simulink model "MPC_RL_H2DF"  (R2023a)
settings: Solver=FixedStepAuto  StartTime=0.0  StopTime=inf  FixedStep=Ts  RelTol=1e-3
model workspace (MAT data in the model file):
  enable_IMEP_noise = 100
  enable_IMEP_offset = 1
values from neighbouring files (symbols this model uses):
  C2C_NMPC = init_C2C_NMPC_H2DF(C2C_NMPC.expdata)    [init_H2DFRL_GRU.m]
  LowerLimit = ([0.17e-3;350;-5;1e-3] - C2C_NMPC.Normalization.controls.mean)./(C2C_NMPC.Normalization.controls.std)    [init_H2DFRL_GRU.m]
  Ts = 0.08    [init_H2DFRL_GRU.m]
  UpperLimit = ([0.5e-3;900;2;5.5e-3] - C2C_NMPC.Normalization.controls.mean)./(C2C_NMPC.Normalization.controls.std)    [init_H2DFRL_GRU.m]
undefined symbols (not defined in the file or in its folder): CA50_offset, DiscIntNeverNeededParam, enable_CA50_noise, enable_CA50_offset, IMEP_offset
libraries: simulink x15, matrix_library x6, dspsigattribs x2, slctrlblks x2, statsLibrary x1, rllib x1
(part 3 of 4)

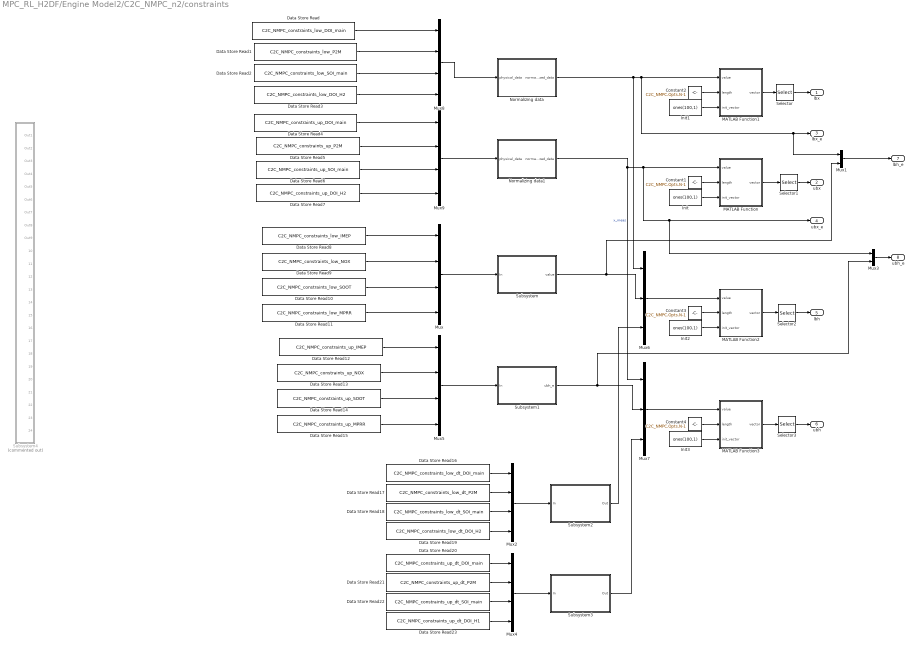
== system MPC_RL_H2DF/Engine Model2/C2C_NMPC_n2/constraints ==
  Constant{1..4} (4 alike) : Constant  Value=C2C_NMPC.Opts.N-1
  Data Store Read : DataStoreRead  DataStoreName=C2C_NMPC_constraints_low_DOI_main  IndexOptions=Index vector (dialog)  Indices=1  OutputSizes=1
  Data Store Read1 : DataStoreRead  DataStoreName=C2C_NMPC_constraints_low_P2M  IndexOptions=Index vector (dialog)  Indices=1  OutputSizes=1
  Data Store Read10 : DataStoreRead  DataStoreName=C2C_NMPC_constraints_low_SOOT  IndexOptions=Index vector (dialog)  Indices=1  OutputSizes=1
  Data Store Read11 : DataStoreRead  DataStoreName=C2C_NMPC_constraints_low_MPRR  IndexOptions=Index vector (dialog)  Indices=1  OutputSizes=1
  Data Store Read12 : DataStoreRead  DataStoreName=C2C_NMPC_constraints_up_IMEP  IndexOptions=Index vector (dialog)  Indices=1  OutputSizes=1
  Data Store Read13 : DataStoreRead  DataStoreName=C2C_NMPC_constraints_up_NOX  IndexOptions=Index vector (dialog)  Indices=1  OutputSizes=1
  Data Store Read14 : DataStoreRead  DataStoreName=C2C_NMPC_constraints_up_SOOT  IndexOptions=Index vector (dialog)  Indices=1  OutputSizes=1
  Data Store Read15 : DataStoreRead  DataStoreName=C2C_NMPC_constraints_up_MPRR  IndexOptions=Index vector (dialog)  Indices=1  OutputSizes=1
  Data Store Read16 : DataStoreRead  DataStoreName=C2C_NMPC_constraints_low_dt_DOI_main  IndexOptions=Index vector (dialog)  Indices=1  OutputSizes=1
  Data Store Read17 : DataStoreRead  DataStoreName=C2C_NMPC_constraints_low_dt_P2M  IndexOptions=Index vector (dialog)  Indices=1  OutputSizes=1
  Data Store Read18 : DataStoreRead  DataStoreName=C2C_NMPC_constraints_low_dt_SOI_main  IndexOptions=Index vector (dialog)  Indices=1  OutputSizes=1
  Data Store Read19 : DataStoreRead  DataStoreName=C2C_NMPC_constraints_low_dt_DOI_H2  IndexOptions=Index vector (dialog)  Indices=1  OutputSizes=1
  Data Store Read2 : DataStoreRead  DataStoreName=C2C_NMPC_constraints_low_SOI_main  IndexOptions=Index vector (dialog)  Indices=1  OutputSizes=1
  Data Store Read20 : DataStoreRead  DataStoreName=C2C_NMPC_constraints_up_dt_DOI_main  IndexOptions=Index vector (dialog)  Indices=1  OutputSizes=1
  Data Store Read21 : DataStoreRead  DataStoreName=C2C_NMPC_constraints_up_dt_P2M  IndexOptions=Index vector (dialog)  Indices=1  OutputSizes=1
  Data Store Read22 : DataStoreRead  DataStoreName=C2C_NMPC_constraints_up_dt_SOI_main  IndexOptions=Index vector (dialog)  Indices=1  OutputSizes=1
  Data Store Read23 : DataStoreRead  DataStoreName=C2C_NMPC_constraints_up_dt_DOI_H1  IndexOptions=Index vector (dialog)  Indices=1  OutputSizes=1
  Data Store Read3 : DataStoreRead  DataStoreName=C2C_NMPC_constraints_low_DOI_H2  IndexOptions=Index vector (dialog)  Indices=1  OutputSizes=1
  Data Store Read4 : DataStoreRead  DataStoreName=C2C_NMPC_constraints_up_DOI_main  IndexOptions=Index vector (dialog)  Indices=1  OutputSizes=1
  Data Store Read5 : DataStoreRead  DataStoreName=C2C_NMPC_constraints_up_P2M  IndexOptions=Index vector (dialog)  Indices=1  OutputSizes=1
  Data Store Read6 : DataStoreRead  DataStoreName=C2C_NMPC_constraints_up_SOI_main  IndexOptions=Index vector (dialog)  Indices=1  OutputSizes=1
  Data Store Read7 : DataStoreRead  DataStoreName=C2C_NMPC_constraints_up_DOI_H2  IndexOptions=Index vector (dialog)  Indices=1  OutputSizes=1
  Data Store Read8 : DataStoreRead  DataStoreName=C2C_NMPC_constraints_low_IMEP  IndexOptions=Index vector (dialog)  Indices=1  OutputSizes=1
  Data Store Read9 : DataStoreRead  DataStoreName=C2C_NMPC_constraints_low_NOX  IndexOptions=Index vector (dialog)  Indices=1  OutputSizes=1
  Init{,1..3} (4 alike) : Constant  Value=ones(100,1)
  MATLAB Function : MATLAB Function  TreatAsAtomicUnit=on
  MATLAB Function1 : MATLAB Function  TreatAsAtomicUnit=on
  MATLAB Function2 : MATLAB Function  TreatAsAtomicUnit=on
  MATLAB Function3 : MATLAB Function  TreatAsAtomicUnit=on
  Mux{,2,4..5,8..9} (6 alike) : Mux
  Mux1 : Mux  Inputs=2
  Mux3 : Mux  Inputs=2
  Mux6 : Mux  Inputs=3
  Mux7 : Mux  Inputs=3
  Normalizing data : Subsystem
  Normalizing data1 : Subsystem
  Selector : Selector  IndexOptions=Index vector (dialog)  Indices=1:((C2C_NMPC.Opts.N-1)*C2C_NMPC.Dims.n_controls)  OutputSizes=1
  Selector1 : Selector  IndexOptions=Index vector (dialog)  Indices=1:((C2C_NMPC.Opts.N-1)*C2C_NMPC.Dims.n_controls)  OutputSizes=1
  Selector2 : Selector  IndexOptions=Index vector (dialog)  Indices=1:((C2C_NMPC.Opts.N)*(C2C_NMPC.Dims.n_outputs + C2C_NMPC.Dims.n_controls +C2C_NMPC.Dims.n_controls))  OutputSizes=1
  Selector3 : Selector  IndexOptions=Index vector (dialog)  Indices=1:((C2C_NMPC.Opts.N)*(C2C_NMPC.Dims.n_outputs + C2C_NMPC.Dims.n_controls +C2C_NMPC.Dims.n_controls))  OutputSizes=1
  Subsystem : Subsystem
  Subsystem1 : Subsystem
  Subsystem2 : Subsystem
  Subsystem3 : Subsystem
  Subsystem4 : Subsystem  Commented=on
  lbx : Outport
  ubx : Outport  Port=2
  lbx_e : Outport  Port=3
  ubx_e : Outport  Port=4
  lbh : Outport  Port=5
  ubh : Outport  Port=6
  lbh_e : Outport  Port=7
  ubh_e : Outport  Port=8
  wires:
  Mux/1 -> Subsystem/1(In)
  Mux5/1 -> Subsystem1/1(In)
  Mux2/1 -> Subsystem2/1(In)
  Mux4/1 -> Subsystem3/1(In)
  Init/1 -> MATLAB Function/3(init_vector)
  Constant1/1 -> MATLAB Function/2(length)
  MATLAB Function/1(vector) -> Selector1/1
  MATLAB Function1/1(vector) -> Selector/1
  Constant2/1 -> MATLAB Function1/2(length)
  Init1/1 -> MATLAB Function1/3(init_vector)
  MATLAB Function2/1(vector) -> Selector2/1
  Constant3/1 -> MATLAB Function2/2(length)
  Init2/1 -> MATLAB Function2/3(init_vector)
  Subsystem3/1(Out) -> Mux7/3
  Mux6/1 -> MATLAB Function2/1(value)
  Normalizing data/1(normalized_data) -> Mux6/1, Mux1/1, lbx_e/1, MATLAB Function1/1(value)
  Subsystem/1(value) -> Mux1/2, Mux6/2
  Subsystem2/1(Out) -> Mux6/3
  MATLAB Function3/1(vector) -> Selector3/1
  Mux7/1 -> MATLAB Function3/1(value)
  Init3/1 -> MATLAB Function3/3(init_vector)
  Constant4/1 -> MATLAB Function3/2(length)
  Data Store Read3/1 -> Mux8/4
  Data Store Read2/1 -> Mux8/3
  Data Store Read1/1 -> Mux8/2
  Data Store Read/1 -> Mux8/1
  Mux8/1 -> Normalizing data/1(physical_data)
  Selector/1 -> lbx/1
  Data Store Read6/1 -> Mux9/3
  Data Store Read5/1 -> Mux9/2
  Data Store Read4/1 -> Mux9/1
  Mux9/1 -> Normalizing data1/1(physical_data)
  Normalizing data1/1(normalized_data) -> Mux7/1, Mux3/1, ubx_e/1, MATLAB Function/1(value)  "x_meas"
  Data Store Read7/1 -> Mux9/4
  Selector1/1 -> ubx/1
  Selector2/1 -> lbh/1
  Selector3/1 -> ubh/1
  Mux1/1 -> lbh_e/1
  Subsystem1/1(ubh_e) -> Mux3/2, Mux7/2
  Mux3/1 -> ubh_e/1
  Data Store Read8/1 -> Mux/1
  Data Store Read9/1 -> Mux/2
  Data Store Read10/1 -> Mux/3
  Data Store Read11/1 -> Mux/4
  Data Store Read12/1 -> Mux5/1
  Data Store Read13/1 -> Mux5/2
  Data Store Read14/1 -> Mux5/3
  Data Store Read15/1 -> Mux5/4
  Data Store Read16/1 -> Mux2/1
  Data Store Read17/1 -> Mux2/2
  Data Store Read18/1 -> Mux2/3
  Data Store Read19/1 -> Mux2/4
  Data Store Read20/1 -> Mux4/1
  Data Store Read21/1 -> Mux4/2
  Data Store Read22/1 -> Mux4/3
  Data Store Read23/1 -> Mux4/4

== system MPC_RL_H2DF/Engine Model2/C2C_NMPC_n2/cost_function_weights ==
  Create Diagonal Matrix : matrix_library/Create Diagonal Matrix
  Create Diagonal Matrix1 : matrix_library/Create Diagonal Matrix
  Create Diagonal Matrix2 : matrix_library/Create Diagonal Matrix
  Data Store Read : DataStoreRead  DataStoreName=C2C_NMPC_IMEP_Weight  IndexOptions=Index vector (dialog)  Indices=1  OutputSizes=1
  Data Store Read1 : DataStoreRead  DataStoreName=C2C_NMPC_NOX_Weight  IndexOptions=Index vector (dialog)  Indices=1  OutputSizes=1
  Data Store Read10 : DataStoreRead  DataStoreName=C2C_NMPC_Delta_SOI_Main_Weight  IndexOptions=Index vector (dialog)  Indices=1  OutputSizes=1
  Data Store Read11 : DataStoreRead  DataStoreName=C2C_NMPC_Delta_DOI_H2_Weight  IndexOptions=Index vector (dialog)  Indices=1  OutputSizes=1
  Data Store Read12 : DataStoreRead  DataStoreName=C2C_NMPC_alpha  IndexOptions=Index vector (dialog)  Indices=1  OutputSizes=1
  Data Store Read13 : DataStoreRead  DataStoreName=C2C_NMPC_beta  IndexOptions=Index vector (dialog)  Indices=1  OutputSizes=1
  Data Store Read14 : DataStoreRead  DataStoreName=C2C_NMPC_gamma  IndexOptions=Index vector (dialog)  Indices=1  OutputSizes=1
  Data Store Read2 : DataStoreRead  DataStoreName=C2C_NMPC_SOOT_Weight  IndexOptions=Index vector (dialog)  Indices=1  OutputSizes=1
  Data Store Read3 : DataStoreRead  DataStoreName=C2C_NMPC_MPRR_Weight  IndexOptions=Index vector (dialog)  Indices=1  OutputSizes=1
  Data Store Read4 : DataStoreRead  DataStoreName=C2C_NMPC_DOI_Main_Weight  IndexOptions=Index vector (dialog)  Indices=1  OutputSizes=1
  Data Store Read5 : DataStoreRead  DataStoreName=C2C_NMPC_P2M_Weight  IndexOptions=Index vector (dialog)  Indices=1  OutputSizes=1
  Data Store Read6 : DataStoreRead  DataStoreName=C2C_NMPC_SOI_Main_Weight  IndexOptions=Index vector (dialog)  Indices=1  OutputSizes=1
  Data Store Read7 : DataStoreRead  DataStoreName=C2C_NMPC_DOI_H2_Weight  IndexOptions=Index vector (dialog)  Indices=1  OutputSizes=1
  Data Store Read8 : DataStoreRead  DataStoreName=C2C_NMPC_Delta_DOI_Main_Weight  IndexOptions=Index vector (dialog)  Indices=1  OutputSizes=1
  Data Store Read9 : DataStoreRead  DataStoreName=C2C_NMPC_Delta_P2M_Weight  IndexOptions=Index vector (dialog)  Indices=1  OutputSizes=1
  Mux : Mux
  Mux2 : Mux
  Mux3 : Mux
  Normalize 0 to 1 : Subsystem
  Product : Product
  Product1 : Product
  Product2 : Product
  alpha : Gain  Commented=on
  beta : Gain  Commented=on  Gain=0.001
  blkdiag Function : MATLAB Function  TreatAsAtomicUnit=on
  blkdiag Function1 : MATLAB Function  TreatAsAtomicUnit=on
  gamma1 : Gain  Commented=on  Gain=2
  cost_W : Outport
  cost_W_e : Outport  Port=2
  wires:
  blkdiag Function/1(y) -> cost_W/1
  Create Diagonal Matrix2/1 -> blkdiag Function/3(u3)
  Product2/1 -> Create Diagonal Matrix2/1
  Create Diagonal Matrix1/1 -> blkdiag Function1/2(u2), blkdiag Function/2(u2)
  Data Store Read7/1 -> Mux3/4
  Data Store Read4/1 -> Mux3/1
  Data Store Read6/1 -> Mux3/3
  Data Store Read5/1 -> Mux3/2
  Mux3/1 -> Product1/1
  Product1/1 -> Create Diagonal Matrix/1
  Product/1 -> Create Diagonal Matrix1/1
  Mux/1 -> Product/1
  Data Store Read1/1 -> Mux/2
  Data Store Read/1 -> Mux/1
  Data Store Read3/1 -> Mux/4
  Data Store Read2/1 -> Mux/3
  Create Diagonal Matrix/1 -> blkdiag Function1/1(u1), blkdiag Function/1(u1)
  Data Store Read8/1 -> Mux2/1
  Data Store Read9/1 -> Mux2/2
  Data Store Read10/1 -> Mux2/3
  Data Store Read11/1 -> Mux2/4
  Data Store Read12/1 -> Product/2
  Data Store Read13/1 -> Product1/2
  Data Store Read14/1 -> Product2/2
  Mux2/1 -> Product2/1
  blkdiag Function1/1(y) -> cost_W_e/1

== system MPC_RL_H2DF/Engine Model2/offset_and_noise/CA50_generation ==
  CA50_in : Inport
  Add : Sum
  Add1 : Sum
  Band-Limited White Noise : simulink/Sources/Band-Limited White Noise  Cov=0.01  Ts=1  seed=[23341]
  Constant1 : Constant  Value=CA50_offset
  Constant2 : Constant  Value=0
  Constant3 : Constant  Value=enable_CA50_noise
  Constant4 : Constant  Value=0
  Constant5 : Constant  Value=enable_CA50_offset
  Switch1 : Switch  Criteria=u2 > Threshold  SaturateOnIntegerOverflow=off  InputSameDT=off
  Switch2 : Switch  Criteria=u2 > Threshold  SaturateOnIntegerOverflow=off  InputSameDT=off
  denormalizing_CA50 : Subsystem
  normalizing_CA50 : Subsystem
  CA50_out : Outport
  wires:
  Add/1 -> Add1/2
  Switch1/1 -> Add1/1
  Constant4/1 -> Switch1/3
  Constant3/1 -> Switch1/2
  Band-Limited White Noise/1 -> Switch1/1
  CA50_in/1 -> denormalizing_CA50/1(CA50_in)
  denormalizing_CA50/1(CA50) -> Add/2
  Switch2/1 -> Add/1
  Constant1/1 -> Switch2/1
  Constant5/1 -> Switch2/2
  Constant2/1 -> Switch2/3
  normalizing_CA50/1(CA50_out) -> CA50_out/1
  Add1/1 -> normalizing_CA50/1(CA50)

== system MPC_RL_H2DF/Engine Model2/offset_and_noise/IMEP_generation ==
  IMEP_in : Inport
  Add : Sum
  Add1 : Sum
  Band-Limited White Noise : simulink/Sources/Band-Limited White Noise  Cov=0.01  Ts=1  seed=[23341]
  Constant1 : Constant  Value=IMEP_offset
  Constant2 : Constant  Value=0
  Constant3 : Constant  Value=enable_IMEP_noise
  Constant4 : Constant  Value=0
  Constant5 : Constant  Value=enable_IMEP_offset
  Switch1 : Switch  Criteria=u2 > Threshold  SaturateOnIntegerOverflow=off  InputSameDT=off
  Switch2 : Switch  Criteria=u2 > Threshold  SaturateOnIntegerOverflow=off  InputSameDT=off
  denormalizing_IMEP : Subsystem
  normalizing_IMEP : Subsystem
  IMEP_out : Outport
  wires:
  Add/1 -> Add1/2
  Switch1/1 -> Add1/1
  Constant4/1 -> Switch1/3
  Constant3/1 -> Switch1/2
  Band-Limited White Noise/1 -> Switch1/1
  IMEP_in/1 -> denormalizing_IMEP/1(IMEP_in)
  denormalizing_IMEP/1(IMEP) -> Add/2
  Switch2/1 -> Add/1
  Constant1/1 -> Switch2/1
  Constant5/1 -> Switch2/2
  Constant2/1 -> Switch2/3
  normalizing_IMEP/1(IMEP_out) -> IMEP_out/1
  Add1/1 -> normalizing_IMEP/1(IMEP)

== system MPC_RL_H2DF/Engine Model2/offset_and_noise1/IMEP_generation ==
  IMEP_in : Inport
  Add : Sum
  Add1 : Sum
  Add2 : Sum  Inputs=+-
  Band-Limited White Noise : simulink/Sources/Band-Limited White Noise  Cov=0.1  Ts=Ts  seed=[23341]
  Constant1 : Constant  Commented=on  Value=IMEP_offset
  Constant2 : Constant  Value=0
  Constant3 : Constant  Value=enable_IMEP_noise
  Constant4 : Constant  Value=0
  Constant5 : Constant  Value=enable_IMEP_offset
  Constant6 : Constant  Value=0
  Display : Display
  Gain : Gain  Gain=10000
  Scope : Scope  NumInputPorts=2
  Scope1 : Scope
  Switch1 : Switch  Criteria=u2 > Threshold  SaturateOnIntegerOverflow=off  InputSameDT=off
  Switch2 : Switch  Criteria=u2 > Threshold  SaturateOnIntegerOverflow=off  InputSameDT=off
  denormalizing_IMEP : Subsystem
  normalizing_IMEP : Subsystem
  IMEP_out : Outport
  wires:
  Add/1 -> Add1/2
  Switch1/1 -> Display/1, Add1/1
  Constant4/1 -> Switch1/3
  Constant3/1 -> Switch1/2
  Band-Limited White Noise/1 -> Gain/1
  denormalizing_IMEP/1(IMEP) -> Add/2
  Switch2/1 -> Add/1
  Constant5/1 -> Switch2/2
  Constant2/1 -> Switch2/3
  normalizing_IMEP/1(IMEP_out) -> IMEP_out/1
  Add1/1 -> Add2/1, Scope/2, normalizing_IMEP/1(IMEP)
  Constant6/1 -> Switch2/1
  Gain/1 -> Switch1/1
  IMEP_in/1 -> Scope/1, Add2/2, denormalizing_IMEP/1(IMEP_in)
  Add2/1 -> Scope1/1

== system MPC_RL_H2DF/Engine Model2/offset_and_noise2/IMEP_generation ==
  IMEP_in : Inport
  Add : Sum
  Add1 : Sum
  Add2 : Sum  Inputs=+-
  Band-Limited White Noise : simulink/Sources/Band-Limited White Noise  Cov=0.1  Ts=Ts  seed=[23341]
  Constant1 : Constant  Commented=on  Value=IMEP_offset
  Constant2 : Constant  Value=0
  Constant3 : Constant  Value=enable_IMEP_noise
  Constant4 : Constant  Value=0
  Constant5 : Constant  Value=enable_IMEP_offset
  Constant6 : Constant  Value=0
  Display : Display
  Gain : Gain  Gain=10000
  Scope : Scope  NumInputPorts=2
  Scope1 : Scope
  Switch1 : Switch  Criteria=u2 > Threshold  SaturateOnIntegerOverflow=off  InputSameDT=off
  Switch2 : Switch  Criteria=u2 > Threshold  SaturateOnIntegerOverflow=off  InputSameDT=off
  denormalizing_IMEP : Subsystem
  normalizing_IMEP : Subsystem
  IMEP_out : Outport
  wires:
  Add/1 -> Add1/2
  Switch1/1 -> Display/1, Add1/1
  Constant4/1 -> Switch1/3
  Constant3/1 -> Switch1/2
  Band-Limited White Noise/1 -> Gain/1
  denormalizing_IMEP/1(IMEP) -> Add/2
  Switch2/1 -> Add/1
  Constant5/1 -> Switch2/2
  Constant2/1 -> Switch2/3
  normalizing_IMEP/1(IMEP_out) -> IMEP_out/1
  Add1/1 -> Add2/1, Scope/2, normalizing_IMEP/1(IMEP)
  Constant6/1 -> Switch2/1
  Gain/1 -> Switch1/1
  IMEP_in/1 -> Scope/1, Add2/2, denormalizing_IMEP/1(IMEP_in)
  Add2/1 -> Scope1/1

== system MPC_RL_H2DF/Engine Model2/offset_and_noise3/IMEP_generation ==
  IMEP_in : Inport
  Add : Sum
  Add1 : Sum
  Add2 : Sum  Inputs=+-
  Band-Limited White Noise : simulink/Sources/Band-Limited White Noise  Cov=0.1  Ts=Ts  seed=[23341]
  Constant1 : Constant  Commented=on  Value=IMEP_offset
  Constant2 : Constant  Value=0
  Constant3 : Constant  Value=enable_IMEP_noise
  Constant4 : Constant  Value=0
  Constant5 : Constant  Value=enable_IMEP_offset
  Constant6 : Constant  Value=0
  Display : Display
  Gain : Gain  Gain=10000
  Scope : Scope  NumInputPorts=2
  Scope1 : Scope
  Switch1 : Switch  Criteria=u2 > Threshold  SaturateOnIntegerOverflow=off  InputSameDT=off
  Switch2 : Switch  Criteria=u2 > Threshold  SaturateOnIntegerOverflow=off  InputSameDT=off
  denormalizing_IMEP : Subsystem
  normalizing_IMEP : Subsystem
  IMEP_out : Outport
  wires:
  Add/1 -> Add1/2
  Switch1/1 -> Display/1, Add1/1
  Constant4/1 -> Switch1/3
  Constant3/1 -> Switch1/2
  Band-Limited White Noise/1 -> Gain/1
  denormalizing_IMEP/1(IMEP) -> Add/2
  Switch2/1 -> Add/1
  Constant5/1 -> Switch2/2
  Constant2/1 -> Switch2/3
  normalizing_IMEP/1(IMEP_out) -> IMEP_out/1
  Add1/1 -> Add2/1, Scope/2, normalizing_IMEP/1(IMEP)
  Constant6/1 -> Switch2/1
  Gain/1 -> Switch1/1
  IMEP_in/1 -> Scope/1, Add2/2, denormalizing_IMEP/1(IMEP_in)
  Add2/1 -> Scope1/1

== system MPC_RL_H2DF/Engine Model2/reference1/Subsystem4 ==
  C2C_NMPC_constraints_low_dt_DOI_H1 : Constant  Value=-1e6
  C2C_NMPC_constraints_low_dt_DOI_main1 : Constant  Value=-1e6
  C2C_NMPC_constraints_low_dt_P2M1 : Constant  Value=-1e6
  C2C_NMPC_constraints_low_dt_SOI_main1 : Constant  Value=-1e6
  C2C_NMPC_constraints_up_dt_DOI_H2 : Constant  Value=1e6
  C2C_NMPC_constraints_up_dt_DOI_main1 : Constant  Value=1e6
  C2C_NMPC_constraints_up_dt_P2M1 : Constant  Value=1e6
  C2C_NMPC_constraints_up_dt_SOI_main1 : Constant  Value=1e6
  Data Store Write16 : DataStoreWrite  DataStoreName=C2C_NMPC_constraints_low_dt_DOI_main  IndexOptions=Index vector (dialog)  Indices=1  OutputSizes=1
  Data Store Write17 : DataStoreWrite  DataStoreName=C2C_NMPC_constraints_low_dt_P2M  IndexOptions=Index vector (dialog)  Indices=1  OutputSizes=1
  Data Store Write18 : DataStoreWrite  DataStoreName=C2C_NMPC_constraints_low_dt_SOI_main  IndexOptions=Index vector (dialog)  Indices=1  OutputSizes=1
  Data Store Write19 : DataStoreWrite  DataStoreName=C2C_NMPC_constraints_low_dt_DOI_H2  IndexOptions=Index vector (dialog)  Indices=1  OutputSizes=1
  Data Store Write20 : DataStoreWrite  DataStoreName=C2C_NMPC_constraints_up_dt_DOI_main  IndexOptions=Index vector (dialog)  Indices=1  OutputSizes=1
  Data Store Write21 : DataStoreWrite  DataStoreName=C2C_NMPC_constraints_up_dt_P2M  IndexOptions=Index vector (dialog)  Indices=1  OutputSizes=1
  Data Store Write22 : DataStoreWrite  DataStoreName=C2C_NMPC_constraints_up_dt_SOI_main  IndexOptions=Index vector (dialog)  Indices=1  OutputSizes=1
  Data Store Write23 : DataStoreWrite  DataStoreName=C2C_NMPC_constraints_up_dt_DOI_H1  IndexOptions=Index vector (dialog)  Indices=1  OutputSizes=1
  wires:
  C2C_NMPC_constraints_up_dt_P2M1/1 -> Data Store Write21/1
  C2C_NMPC_constraints_low_dt_SOI_main1/1 -> Data Store Write18/1
  C2C_NMPC_constraints_up_dt_DOI_main1/1 -> Data Store Write20/1
  C2C_NMPC_constraints_low_dt_P2M1/1 -> Data Store Write17/1
  C2C_NMPC_constraints_up_dt_SOI_main1/1 -> Data Store Write22/1
  C2C_NMPC_constraints_low_dt_DOI_main1/1 -> Data Store Write16/1
  C2C_NMPC_constraints_low_dt_DOI_H1/1 -> Data Store Write19/1
  C2C_NMPC_constraints_up_dt_DOI_H2/1 -> Data Store Write23/1

== system MPC_RL_H2DF/Engine Model2/results/denormalizing physical controls and outputs ==
  IMEP_norm : Inport
  NOX_norm : Inport  Port=2
  soot_norm : Inport  Port=3
  MPRR_norm : Inport  Port=4
  DOI_main_norm : Inport  Port=5
  SOI_pre_norm : Inport  Port=6
  SOI_main_norm : Inport  Port=7
  DOI_H2_norm : Inport  Port=8
  Constant : Constant  Value=C2C_NMPC.Normalization.outputs.mean(1)
  Constant1 : Constant  Value=C2C_NMPC.Normalization.controls.mean(4)
  Constant3 : Constant  Value=C2C_NMPC.Normalization.outputs.mean(2)
  Constant4 : Constant  Value=C2C_NMPC.Normalization.outputs.mean(3)
  Constant5 : Constant  Value=C2C_NMPC.Normalization.outputs.mean(4)
  Constant6 : Constant  Value=C2C_NMPC.Normalization.controls.mean(1)
  Constant7 : Constant  Value=C2C_NMPC.Normalization.controls.mean(2)
  Constant8 : Constant  Value=C2C_NMPC.Normalization.controls.mean(3)
  Gain : Gain  Gain=C2C_NMPC.Normalization.outputs.std(1)
  Gain1 : Gain  Gain=C2C_NMPC.Normalization.controls.std(4)
  Gain3 : Gain  Gain=C2C_NMPC.Normalization.outputs.std(2)
  Gain4 : Gain  Gain=C2C_NMPC.Normalization.outputs.std(3)
  Gain5 : Gain  Gain=C2C_NMPC.Normalization.outputs.std(4)
  Gain6 : Gain  Gain=C2C_NMPC.Normalization.controls.std(1)
  Gain7 : Gain  Gain=C2C_NMPC.Normalization.controls.std(2)
  Gain8 : Gain  Gain=C2C_NMPC.Normalization.controls.std(3)
  Sum{1,3..8,10} (8 alike) : Sum  Inputs=|++
  IMEP : Outport
  NOX : Outport  Port=2
  soot : Outport  Port=3
  MPRR : Outport  Port=4
  DOI_main : Outport  Port=5
  SOI_pre : Outport  Port=6
  SOI_main : Outport  Port=7
  DOI_H2 : Outport  Port=8
  wires:
  Gain4/1 -> Sum4/1
  Constant3/1 -> Sum3/2
  Constant4/1 -> Sum4/2
  Gain3/1 -> Sum3/1
  Constant5/1 -> Sum5/2
  Gain5/1 -> Sum5/1
  Constant/1 -> Sum6/2
  Sum3/1 -> NOX/1
  NOX_norm/1 -> Gain3/1
  Sum5/1 -> MPRR/1
  Gain/1 -> Sum6/1
  IMEP_norm/1 -> Gain/1
  Sum6/1 -> IMEP/1
  MPRR_norm/1 -> Gain5/1
  Sum4/1 -> soot/1
  soot_norm/1 -> Gain4/1
  Constant7/1 -> Sum8/2
  Gain8/1 -> Sum10/1
  Constant6/1 -> Sum7/2
  Gain7/1 -> Sum8/1
  Sum10/1 -> SOI_main/1
  DOI_main_norm/1 -> Gain6/1
  Sum7/1 -> DOI_main/1
  Gain6/1 -> Sum7/1
  Sum8/1 -> SOI_pre/1
  Constant8/1 -> Sum10/2
  SOI_main_norm/1 -> Gain8/1
  SOI_pre_norm/1 -> Gain7/1
  DOI_H2_norm/1 -> Gain1/1
  Constant1/1 -> Sum1/2
  Gain1/1 -> Sum1/1
  Sum1/1 -> DOI_H2/1

== system MPC_RL_H2DF/Engine Model2/results/denormalizing reference ==
  IMEP_norm : Inport
  NOX_norm : Inport  Port=2
  soot_norm : Inport  Port=3
  MPRR_norm : Inport  Port=4
  Constant : Constant  Value=C2C_NMPC.Normalization.outputs.mean(1)
  Constant1 : Constant  Value=C2C_NMPC.Normalization.outputs.mean(2)
  Constant2 : Constant  Value=C2C_NMPC.Normalization.outputs.mean(3)
  Constant3 : Constant  Value=C2C_NMPC.Normalization.outputs.mean(4)
  Gain : Gain  Gain=C2C_NMPC.Normalization.outputs.std(1)
  Gain1 : Gain  Gain=C2C_NMPC.Normalization.outputs.std(2)
  Gain2 : Gain  Gain=C2C_NMPC.Normalization.outputs.std(3)
  Gain3 : Gain  Gain=C2C_NMPC.Normalization.outputs.std(4)
  Sum{1..3,5} (4 alike) : Sum  Inputs=|++
  IMEP : Outport
  NOX : Outport  Port=2
  soot : Outport  Port=3
  MPRR : Outport  Port=4
  wires:
  Gain/1 -> Sum5/1
  IMEP_norm/1 -> Gain/1
  Constant/1 -> Sum5/2
  Sum5/1 -> IMEP/1
  Gain1/1 -> Sum1/1
  Constant1/1 -> Sum1/2
  NOX_norm/1 -> Gain1/1
  Sum1/1 -> NOX/1
  Gain2/1 -> Sum2/1
  Constant2/1 -> Sum2/2
  soot_norm/1 -> Gain2/1
  Sum2/1 -> soot/1
  Gain3/1 -> Sum3/1
  Constant3/1 -> Sum3/2
  MPRR_norm/1 -> Gain3/1
  Sum3/1 -> MPRR/1

== system MPC_RL_H2DF/Engine Model2/results1/denormalizing physical controls and outputs ==
  IMEP_norm : Inport
  NOX_norm : Inport  Port=2
  soot_norm : Inport  Port=3
  MPRR_norm : Inport  Port=4
  DOI_main_norm : Inport  Port=5
  SOI_pre_norm : Inport  Port=6
  SOI_main_norm : Inport  Port=7
  DOI_H2_norm : Inport  Port=8
  Constant : Constant  Value=C2C_NMPC.Normalization.outputs.mean(1)
  Constant1 : Constant  Value=C2C_NMPC.Normalization.controls.mean(4)
  Constant3 : Constant  Value=C2C_NMPC.Normalization.outputs.mean(2)
  Constant4 : Constant  Value=C2C_NMPC.Normalization.outputs.mean(3)
  Constant5 : Constant  Value=C2C_NMPC.Normalization.outputs.mean(4)
  Constant6 : Constant  Value=C2C_NMPC.Normalization.controls.mean(1)
  Constant7 : Constant  Value=C2C_NMPC.Normalization.controls.mean(2)
  Constant8 : Constant  Value=C2C_NMPC.Normalization.controls.mean(3)
  Gain : Gain  Gain=C2C_NMPC.Normalization.outputs.std(1)
  Gain1 : Gain  Gain=C2C_NMPC.Normalization.controls.std(4)
  Gain3 : Gain  Gain=C2C_NMPC.Normalization.outputs.std(2)
  Gain4 : Gain  Gain=C2C_NMPC.Normalization.outputs.std(3)
  Gain5 : Gain  Gain=C2C_NMPC.Normalization.outputs.std(4)
  Gain6 : Gain  Gain=C2C_NMPC.Normalization.controls.std(1)
  Gain7 : Gain  Gain=C2C_NMPC.Normalization.controls.std(2)
  Gain8 : Gain  Gain=C2C_NMPC.Normalization.controls.std(3)
  Sum{1,3..8,10} (8 alike) : Sum  Inputs=|++
  IMEP : Outport
  NOX : Outport  Port=2
  soot : Outport  Port=3
  MPRR : Outport  Port=4
  DOI_main : Outport  Port=5
  SOI_pre : Outport  Port=6
  SOI_main : Outport  Port=7
  DOI_H2 : Outport  Port=8
  wires:
  Gain4/1 -> Sum4/1
  Constant3/1 -> Sum3/2
  Constant4/1 -> Sum4/2
  Gain3/1 -> Sum3/1
  Constant5/1 -> Sum5/2
  Gain5/1 -> Sum5/1
  Constant/1 -> Sum6/2
  Sum3/1 -> NOX/1
  NOX_norm/1 -> Gain3/1
  Sum5/1 -> MPRR/1
  Gain/1 -> Sum6/1
  IMEP_norm/1 -> Gain/1
  Sum6/1 -> IMEP/1
  MPRR_norm/1 -> Gain5/1
  Sum4/1 -> soot/1
  soot_norm/1 -> Gain4/1
  Constant7/1 -> Sum8/2
  Gain8/1 -> Sum10/1
  Constant6/1 -> Sum7/2
  Gain7/1 -> Sum8/1
  Sum10/1 -> SOI_main/1
  DOI_main_norm/1 -> Gain6/1
  Sum7/1 -> DOI_main/1
  Gain6/1 -> Sum7/1
  Sum8/1 -> SOI_pre/1
  Constant8/1 -> Sum10/2
  SOI_main_norm/1 -> Gain8/1
  SOI_pre_norm/1 -> Gain7/1
  DOI_H2_norm/1 -> Gain1/1
  Constant1/1 -> Sum1/2
  Gain1/1 -> Sum1/1
  Sum1/1 -> DOI_H2/1

== system MPC_RL_H2DF/Engine Model2/results1/denormalizing reference ==
  IMEP_norm : Inport
  NOX_norm : Inport  Port=2
  soot_norm : Inport  Port=3
  MPRR_norm : Inport  Port=4
  Constant : Constant  Value=C2C_NMPC.Normalization.outputs.mean(1)
  Constant1 : Constant  Value=C2C_NMPC.Normalization.outputs.mean(2)
  Constant2 : Constant  Value=C2C_NMPC.Normalization.outputs.mean(3)
  Constant3 : Constant  Value=C2C_NMPC.Normalization.outputs.mean(4)
  Gain : Gain  Gain=C2C_NMPC.Normalization.outputs.std(1)
  Gain1 : Gain  Gain=C2C_NMPC.Normalization.outputs.std(2)
  Gain2 : Gain  Gain=C2C_NMPC.Normalization.outputs.std(3)
  Gain3 : Gain  Gain=C2C_NMPC.Normalization.outputs.std(4)
  Sum{1..3,5} (4 alike) : Sum  Inputs=|++
  IMEP : Outport
  NOX : Outport  Port=2
  soot : Outport  Port=3
  MPRR : Outport  Port=4
  wires:
  Gain/1 -> Sum5/1
  IMEP_norm/1 -> Gain/1
  Constant/1 -> Sum5/2
  Sum5/1 -> IMEP/1
  Gain1/1 -> Sum1/1
  Constant1/1 -> Sum1/2
  NOX_norm/1 -> Gain1/1
  Sum1/1 -> NOX/1
  Gain2/1 -> Sum2/1
  Constant2/1 -> Sum2/2
  soot_norm/1 -> Gain2/1
  Sum2/1 -> soot/1
  Gain3/1 -> Sum3/1
  Constant3/1 -> Sum3/2
  MPRR_norm/1 -> Gain3/1
  Sum3/1 -> MPRR/1

== system MPC_RL_H2DF/Engine Model2/results2/denormalizing physical controls and outputs ==
  IMEP_norm : Inport
  NOX_norm : Inport  Port=2
  soot_norm : Inport  Port=3
  MPRR_norm : Inport  Port=4
  DOI_main_norm : Inport  Port=5
  SOI_pre_norm : Inport  Port=6
  SOI_main_norm : Inport  Port=7
  DOI_H2_norm : Inport  Port=8
  Constant : Constant  Value=C2C_NMPC.Normalization.outputs.mean(1)
  Constant1 : Constant  Value=C2C_NMPC.Normalization.controls.mean(4)
  Constant3 : Constant  Value=C2C_NMPC.Normalization.outputs.mean(2)
  Constant4 : Constant  Value=C2C_NMPC.Normalization.outputs.mean(3)
  Constant5 : Constant  Value=C2C_NMPC.Normalization.outputs.mean(4)
  Constant6 : Constant  Value=C2C_NMPC.Normalization.controls.mean(1)
  Constant7 : Constant  Value=C2C_NMPC.Normalization.controls.mean(2)
  Constant8 : Constant  Value=C2C_NMPC.Normalization.controls.mean(3)
  Gain : Gain  Gain=C2C_NMPC.Normalization.outputs.std(1)
  Gain1 : Gain  Gain=C2C_NMPC.Normalization.controls.std(4)
  Gain3 : Gain  Gain=C2C_NMPC.Normalization.outputs.std(2)
  Gain4 : Gain  Gain=C2C_NMPC.Normalization.outputs.std(3)
  Gain5 : Gain  Gain=C2C_NMPC.Normalization.outputs.std(4)
  Gain6 : Gain  Gain=C2C_NMPC.Normalization.controls.std(1)
  Gain7 : Gain  Gain=C2C_NMPC.Normalization.controls.std(2)
  Gain8 : Gain  Gain=C2C_NMPC.Normalization.controls.std(3)
  Sum{1,3..8,10} (8 alike) : Sum  Inputs=|++
  IMEP : Outport
  NOX : Outport  Port=2
  soot : Outport  Port=3
  MPRR : Outport  Port=4
  DOI_main : Outport  Port=5
  SOI_pre : Outport  Port=6
  SOI_main : Outport  Port=7
  DOI_H2 : Outport  Port=8
  wires:
  Gain4/1 -> Sum4/1
  Constant3/1 -> Sum3/2
  Constant4/1 -> Sum4/2
  Gain3/1 -> Sum3/1
  Constant5/1 -> Sum5/2
  Gain5/1 -> Sum5/1
  Constant/1 -> Sum6/2
  Sum3/1 -> NOX/1
  NOX_norm/1 -> Gain3/1
  Sum5/1 -> MPRR/1
  Gain/1 -> Sum6/1
  IMEP_norm/1 -> Gain/1
  Sum6/1 -> IMEP/1
  MPRR_norm/1 -> Gain5/1
  Sum4/1 -> soot/1
  soot_norm/1 -> Gain4/1
  Constant7/1 -> Sum8/2
  Gain8/1 -> Sum10/1
  Constant6/1 -> Sum7/2
  Gain7/1 -> Sum8/1
  Sum10/1 -> SOI_main/1
  DOI_main_norm/1 -> Gain6/1
  Sum7/1 -> DOI_main/1
  Gain6/1 -> Sum7/1
  Sum8/1 -> SOI_pre/1
  Constant8/1 -> Sum10/2
  SOI_main_norm/1 -> Gain8/1
  SOI_pre_norm/1 -> Gain7/1
  DOI_H2_norm/1 -> Gain1/1
  Constant1/1 -> Sum1/2
  Gain1/1 -> Sum1/1
  Sum1/1 -> DOI_H2/1

== system MPC_RL_H2DF/Engine Model2/results2/denormalizing reference ==
  IMEP_norm : Inport
  NOX_norm : Inport  Port=2
  soot_norm : Inport  Port=3
  MPRR_norm : Inport  Port=4
  Constant : Constant  Value=C2C_NMPC.Normalization.outputs.mean(1)
  Constant1 : Constant  Value=C2C_NMPC.Normalization.outputs.mean(2)
  Constant2 : Constant  Value=C2C_NMPC.Normalization.outputs.mean(3)
  Constant3 : Constant  Value=C2C_NMPC.Normalization.outputs.mean(4)
  Gain : Gain  Gain=C2C_NMPC.Normalization.outputs.std(1)
  Gain1 : Gain  Gain=C2C_NMPC.Normalization.outputs.std(2)
  Gain2 : Gain  Gain=C2C_NMPC.Normalization.outputs.std(3)
  Gain3 : Gain  Gain=C2C_NMPC.Normalization.outputs.std(4)
  Sum{1..3,5} (4 alike) : Sum  Inputs=|++
  IMEP : Outport
  NOX : Outport  Port=2
  soot : Outport  Port=3
  MPRR : Outport  Port=4
  wires:
  Gain/1 -> Sum5/1
  IMEP_norm/1 -> Gain/1
  Constant/1 -> Sum5/2
  Sum5/1 -> IMEP/1
  Gain1/1 -> Sum1/1
  Constant1/1 -> Sum1/2
  NOX_norm/1 -> Gain1/1
  Sum1/1 -> NOX/1
  Gain2/1 -> Sum2/1
  Constant2/1 -> Sum2/2
  soot_norm/1 -> Gain2/1
  Sum2/1 -> soot/1
  Gain3/1 -> Sum3/1
  Constant3/1 -> Sum3/2
  MPRR_norm/1 -> Gain3/1
  Sum3/1 -> MPRR/1

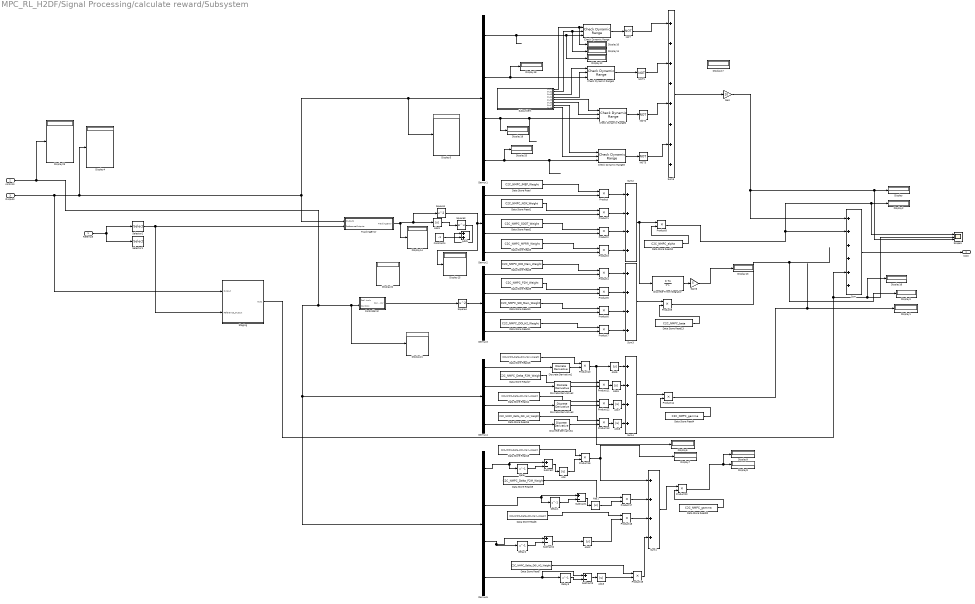
== system MPC_RL_H2DF/Signal Processing/calculate reward/Subsystem ==
  Refernce : Inport
  controls : Inport  Port=2
  Outputs : Inport  Port=3
  Abs{,1..3,5..9} (9 alike) : Abs  SaturateOnIntegerOverflow=off
  Add1 : Sum
  Check Dynamic Range{,1..3} (4 alike) : simulink/Model Verification/Check  Dynamic Range  Description=min < u < max  enabled=off  stopWhenAssertionFail=off  export=on  icon=graphic
  Constant4 : Constant  Value=-1
  ControlError : Subsystem
  Data Store Read : DataStoreRead  DataStoreName=C2C_NMPC_IMEP_Weight  IndexOptions=Index vector (dialog)  Indices=1  OutputSizes=1
  Data Store Read1 : DataStoreRead  DataStoreName=C2C_NMPC_NOX_Weight  IndexOptions=Index vector (dialog)  Indices=1  OutputSizes=1
  Data Store Read10 : DataStoreRead  DataStoreName=C2C_NMPC_SOI_Main_Weight  IndexOptions=Index vector (dialog)  Indices=1  OutputSizes=1
  Data Store Read11 : DataStoreRead  DataStoreName=C2C_NMPC_DOI_H2_Weight  IndexOptions=Index vector (dialog)  Indices=1  OutputSizes=1
  Data Store Read12 : DataStoreRead  DataStoreName=C2C_NMPC_alpha  IndexOptions=Index vector (dialog)  Indices=1  OutputSizes=1
  Data Store Read13 : DataStoreRead  DataStoreName=C2C_NMPC_beta  IndexOptions=Index vector (dialog)  Indices=1  OutputSizes=1
  Data Store Read14 : DataStoreRead  DataStoreName=C2C_NMPC_Delta_SOI_Main_Weight  IndexOptions=Index vector (dialog)  Indices=1  OutputSizes=1
  Data Store Read15 : DataStoreRead  DataStoreName=C2C_NMPC_Delta_DOI_H2_Weight  IndexOptions=Index vector (dialog)  Indices=1  OutputSizes=1
  Data Store Read16 : DataStoreRead  DataStoreName=C2C_NMPC_Delta_DOI_Main_Weight  IndexOptions=Index vector (dialog)  Indices=1  OutputSizes=1
  Data Store Read17 : DataStoreRead  DataStoreName=C2C_NMPC_Delta_P2M_Weight  IndexOptions=Index vector (dialog)  Indices=1  OutputSizes=1
  Data Store Read18 : DataStoreRead  DataStoreName=C2C_NMPC_Delta_DOI_Main_Weight  IndexOptions=Index vector (dialog)  Indices=1  OutputSizes=1
  Data Store Read19 : DataStoreRead  DataStoreName=C2C_NMPC_Delta_P2M_Weight  IndexOptions=Index vector (dialog)  Indices=1  OutputSizes=1
  Data Store Read2 : DataStoreRead  DataStoreName=C2C_NMPC_SOOT_Weight  IndexOptions=Index vector (dialog)  Indices=1  OutputSizes=1
  Data Store Read20 : DataStoreRead  DataStoreName=C2C_NMPC_gamma  IndexOptions=Index vector (dialog)  Indices=1  OutputSizes=1
  Data Store Read3 : DataStoreRead  DataStoreName=C2C_NMPC_MPRR_Weight  IndexOptions=Index vector (dialog)  Indices=1  OutputSizes=1
  Data Store Read4 : DataStoreRead  DataStoreName=C2C_NMPC_gamma  IndexOptions=Index vector (dialog)  Indices=1  OutputSizes=1
  Data Store Read6 : DataStoreRead  DataStoreName=C2C_NMPC_Delta_SOI_Main_Weight  IndexOptions=Index vector (dialog)  Indices=1  OutputSizes=1
  Data Store Read7 : DataStoreRead  DataStoreName=C2C_NMPC_Delta_DOI_H2_Weight  IndexOptions=Index vector (dialog)  Indices=1  OutputSizes=1
  Data Store Read8 : DataStoreRead  DataStoreName=C2C_NMPC_DOI_Main_Weight  IndexOptions=Index vector (dialog)  Indices=1  OutputSizes=1
  Data Store Read9 : DataStoreRead  DataStoreName=C2C_NMPC_P2M_Weight  IndexOptions=Index vector (dialog)  Indices=1  OutputSizes=1
  Delay{,1..3} (4 alike) : Delay  DelayLength=1
  Demux{1..5} (5 alike) : Demux
  Discrete Derivative{1..4} (4 alike) : simulink/Discrete/Discrete Derivative  gainval=1.0  ICPrevScaledInput=0.0  OutMin=[]  OutMax=[]  OutDataType=fixdt(1, 16)  OutScaling=2^-10  DoSatur=off
  Discrete-Time Integrator : DiscreteIntegrator  SampleTime=-1  ICPrevOutput=DiscIntNeverNeededParam  ICPrevScaledInput=DiscIntNeverNeededParam
  Display{,1..23} (24 alike) : Display
  Gain : Gain  Gain=20
  Gain6 : Gain  Gain=5
  NOT{,1..3} (4 alike) : Logic  Operator=NOT  IconShape=distinctive  AllPortsSameDT=off  OutDataTypeStr=boolean
  Product{,1..14,16..20} (20 alike) : Product
  Scope1 : Scope  NumInputPorts=3
  Selector1 : Selector  IndexOptions=Index vector (dialog)  Indices=[5:8]  OutputSizes=1
  Selector2 : Selector  IndexOptions=Index vector (dialog)  Indices=[1:4]  OutputSizes=1
  Square1 : Math  Operator=square  SignedPower=on
  Square3 : Math  SignedPower=on
  Square4 : Math  Operator=square  SignedPower=on
  Staging : Subsystem
  Subsystem : Subsystem
  Subtract{,1..3} (4 alike) : Sum  Inputs=+-
  Sum : Sum  Inputs=++++++
  Sum{1..4} (4 alike) : Sum  Inputs=++++
  Sum5 : Sum  Inputs=++++++++
  TrackingError : Subsystem
  Cost : Outport  VectorParamsAs1DForOutWhenUnconnected=off
  wires:
  Sum/1 -> Cost/1
  Outputs/1 -> Display5/1, Demux1/1, TrackingError/1(Outputs), Display4/1, Staging/1(Output)
  Data Store Read/1 -> Product/1
  Demux2/1 -> Product/2
  Demux2/2 -> Product1/2
  Data Store Read1/1 -> Product1/1
  Demux2/3 -> Product2/2
  Data Store Read2/1 -> Product2/1
  Demux2/4 -> Product3/2
  Data Store Read3/1 -> Product3/1
  Product2/1 -> Sum2/3
  Product1/1 -> Sum2/2
  Product/1 -> Sum2/1
  Product3/1 -> Sum2/4
  TrackingError/1(TrackingError) -> Square1/1, Abs9/1, Display14/1
  Product4/1 -> Sum3/1
  Data Store Read10/1 -> Product6/1
  Product7/1 -> Sum3/4
  Product5/1 -> Sum3/2
  Demux3/3 -> Product6/2
  Data Store Read8/1 -> Product4/1
  Demux3/4 -> Product7/2
  ControlError/1(ControlError) -> Square4/1
  Data Store Read9/1 -> Product5/1
  Product6/1 -> Sum3/3
  Demux3/1 -> Product4/2
  Demux3/2 -> Product5/2
  Data Store Read11/1 -> Product7/1
  Sum2/1 -> Discrete-Time Integrator/1, Product8/1
  Data Store Read12/1 -> Product8/2
  Sum3/1 -> Product9/1
  Data Store Read13/1 -> Product9/2
  Square4/1 -> Demux3/1
  Data Store Read17/1 -> Product11/1
  Data Store Read15/1 -> Product13/1
  Demux4/2 -> Discrete Derivative2/1
  Demux4/1 -> Discrete Derivative1/1
  Product12/1 -> Abs7/1
  Product10/1 -> Display6/1, Abs5/1
  Product13/1 -> Abs8/1
  Demux4/4 -> Discrete Derivative4/1
  Demux4/3 -> Discrete Derivative3/1
  Data Store Read16/1 -> Product10/1
  Data Store Read14/1 -> Product12/1
  Product11/1 -> Abs6/1
  Discrete Derivative1/1 -> Product10/2
  Discrete Derivative2/1 -> Product11/2
  Discrete Derivative3/1 -> Product12/2
  Discrete Derivative4/1 -> Product13/2
  Data Store Read4/1 -> Product14/2
  Sum4/1 -> Product14/1
  Demux1/1 -> Display12/1, Check Dynamic Range/3
  Check Dynamic Range/1 -> NOT/1
  Check Dynamic Range1/1 -> NOT1/1
  Check Dynamic Range2/1 -> NOT2/1
  Check Dynamic Range3/1 -> NOT3/1
  Sum5/1 -> Gain/1
  Product8/1 -> Scope1/1, Display2/1, Sum/2
  Product20/1 -> Display9/1, Display8/1
  Product9/1 -> Display3/1
  Refernce/1 -> Selector2/1, Selector1/1
  Selector2/1 -> Staging/2(Reference_Output), TrackingError/2(ReferenceOutputs)
  Subsystem/1(Out1) -> Display10/1, Check Dynamic Range/1
  Subsystem/2(Out2) -> Display11/1, Check Dynamic Range/2
  Subsystem/3(Out3) -> Check Dynamic Range1/1
  Subsystem/4(Out4) -> Check Dynamic Range1/2
  Subsystem/5(Out5) -> Check Dynamic Range2/1
  Subsystem/6(Out6) -> Check Dynamic Range2/2
  Subsystem/7(Out7) -> Check Dynamic Range3/1
  Subsystem/8(Out8) -> Check Dynamic Range3/2
  Product19/1 -> Sum1/4
  Product16/1 -> Display7/1, Sum1/1
  Abs/1 -> Product16/2
  Product18/1 -> Sum1/3
  Demux5/1 -> Subtract/1, Delay/1
  Product17/1 -> Sum1/2
  Data Store Read7/1 -> Product19/1
  Data Store Read6/1 -> Product18/1
  Abs3/1 -> Product19/2
  Data Store Read19/1 -> Product17/1
  Data Store Read18/1 -> Product16/1
  Sum1/1 -> Product20/1
  Data Store Read20/1 -> Product20/2
  Delay/1 -> Subtract/2
  Subtract/1 -> Abs/1
  Subtract1/1 -> Abs1/1
  Delay1/1 -> Subtract1/2
  Demux5/2 -> Subtract1/1, Delay1/1
  Abs1/1 -> Product17/2
  Demux5/3 -> Subtract2/1, Delay2/1
  Delay2/1 -> Subtract2/2
  Subtract2/1 -> Abs2/1
  Abs2/1 -> Product18/2
  Demux5/4 -> Subtract3/1, Delay3/1
  Delay3/1 -> Subtract3/2
  Subtract3/1 -> Abs3/1
  Product14/1 -> Display1/1
  controls/1 -> Display23/1, Demux4/1, Demux5/1, Display21/1, ControlError/2(Controls)
  NOT/1 -> Sum5/1
  NOT1/1 -> Sum5/3
  NOT2/1 -> Sum5/5
  NOT3/1 -> Sum5/7
  Abs5/1 -> Sum4/1
  Abs6/1 -> Sum4/2
  Abs7/1 -> Sum4/3
  Abs8/1 -> Sum4/4
  Gain/1 -> Sum/1, Scope1/3, Display/1
  Discrete-Time Integrator/1 -> Gain6/1
  Gain6/1 -> Display13/1
  Constant4/1 -> Add1/2
  Abs9/1 -> Square3/1
  Square3/1 -> Add1/1
  Square1/1 -> Display15/1, Demux2/1
  ? -> ?
  ? -> Display17/1, Sum5/2
  Demux1/2 -> Display18/1, Check Dynamic Range1/3
  Demux1/3 -> Check Dynamic Range2/3, Display19/1
  ? -> Sum5/6
  Demux1/4 -> Check Dynamic Range3/3, Display20/1
  Staging/1(Out1) -> Scope1/2, Display16/1, Sum/5

== system MPC_RL_H2DF/Engine Model2/C2C_NMPC_n1/constraints/Normalizing data ==
  physical_data : Inport
  Constant1 : Constant  Value=C2C_NMPC.Normalization.controls.mean(2)
  Constant2 : Constant  Value=C2C_NMPC.Normalization.controls.mean(3)
  Constant3 : Constant  Value=C2C_NMPC.Normalization.controls.mean(1)
  Constant4 : Constant  Value=C2C_NMPC.Normalization.controls.mean(4)
  Gain1 : Gain  Gain=1/C2C_NMPC.Normalization.controls.std(2)
  Gain2 : Gain  Gain=1/C2C_NMPC.Normalization.controls.std(3)
  Gain3 : Gain  Gain=1/C2C_NMPC.Normalization.controls.std(4)
  Gain4 : Gain  Gain=1/C2C_NMPC.Normalization.controls.std(1)
  Mux : Mux
  Selector : Selector  IndexOptions=Index vector (dialog)  Indices=[2]  OutputSizes=1
  Selector1 : Selector  IndexOptions=Index vector (dialog)  Indices=[1]  OutputSizes=1
  Selector2 : Selector  IndexOptions=Index vector (dialog)  Indices=[3]  OutputSizes=1
  Selector3 : Selector  IndexOptions=Index vector (dialog)  Indices=[4]  OutputSizes=1
  Sum{1..4} (4 alike) : Sum  Inputs=|+-
  normalized_data : Outport
  wires:
  Constant3/1 -> Sum4/2
  Selector2/1 -> Sum3/1
  Constant2/1 -> Sum3/2
  Sum4/1 -> Gain4/1
  Sum3/1 -> Gain2/1
  Selector/1 -> Sum2/1
  Constant1/1 -> Sum2/2
  Sum2/1 -> Gain1/1
  Sum1/1 -> Gain3/1
  Constant4/1 -> Sum1/2
  Selector3/1 -> Sum1/1
  Selector1/1 -> Sum4/1
  Gain4/1 -> Mux/1
  Gain1/1 -> Mux/2
  Gain2/1 -> Mux/3
  Gain3/1 -> Mux/4
  Mux/1 -> normalized_data/1
  physical_data/1 -> Selector1/1, Selector/1, Selector3/1, Selector2/1

== system MPC_RL_H2DF/Engine Model2/C2C_NMPC_n1/constraints/Normalizing data1 ==
  physical_data : Inport
  Constant1 : Constant  Value=C2C_NMPC.Normalization.controls.mean(2)
  Constant2 : Constant  Value=C2C_NMPC.Normalization.controls.mean(3)
  Constant3 : Constant  Value=C2C_NMPC.Normalization.controls.mean(1)
  Constant4 : Constant  Value=C2C_NMPC.Normalization.controls.mean(4)
  Gain1 : Gain  Gain=1/C2C_NMPC.Normalization.controls.std(2)
  Gain2 : Gain  Gain=1/C2C_NMPC.Normalization.controls.std(3)
  Gain3 : Gain  Gain=1/C2C_NMPC.Normalization.controls.std(4)
  Gain4 : Gain  Gain=1/C2C_NMPC.Normalization.controls.std(1)
  Mux : Mux
  Selector : Selector  IndexOptions=Index vector (dialog)  Indices=[2]  OutputSizes=1
  Selector1 : Selector  IndexOptions=Index vector (dialog)  Indices=[1]  OutputSizes=1
  Selector2 : Selector  IndexOptions=Index vector (dialog)  Indices=[3]  OutputSizes=1
  Selector3 : Selector  IndexOptions=Index vector (dialog)  Indices=[4]  OutputSizes=1
  Sum{1..4} (4 alike) : Sum  Inputs=|+-
  normalized_data : Outport
  wires:
  Constant3/1 -> Sum4/2
  Selector2/1 -> Sum3/1
  Constant2/1 -> Sum3/2
  Sum4/1 -> Gain4/1
  Sum3/1 -> Gain2/1
  Selector/1 -> Sum2/1
  Constant1/1 -> Sum2/2
  Sum2/1 -> Gain1/1
  Sum1/1 -> Gain3/1
  Constant4/1 -> Sum1/2
  Selector3/1 -> Sum1/1
  Selector1/1 -> Sum4/1
  Gain4/1 -> Mux/1
  Gain1/1 -> Mux/2
  Gain2/1 -> Mux/3
  Gain3/1 -> Mux/4
  Mux/1 -> normalized_data/1
  physical_data/1 -> Selector1/1, Selector/1, Selector3/1, Selector2/1

== system MPC_RL_H2DF/Engine Model2/C2C_NMPC_n1/constraints/Subsystem ==
  In : Inport
  Constant : Constant  Value=C2C_NMPC.Normalization.outputs.mean(1)
  Constant1 : Constant  Value=C2C_NMPC.Normalization.outputs.mean(2)
  Constant2 : Constant  Value=C2C_NMPC.Normalization.outputs.mean(3)
  Constant3 : Constant  Value=C2C_NMPC.Normalization.outputs.mean(4)
  Demux : Demux
  Gain : Gain  Gain=1/C2C_NMPC.Normalization.outputs.std(1)
  Gain1 : Gain  Gain=1/C2C_NMPC.Normalization.outputs.std(2)
  Gain2 : Gain  Gain=1/C2C_NMPC.Normalization.outputs.std(3)
  Gain3 : Gain  Gain=1/C2C_NMPC.Normalization.outputs.std(4)
  Mux : Mux
  Sum{1..3,5} (4 alike) : Sum  Inputs=|+-
  value : Outport
  wires:
  Constant/1 -> Sum5/2
  Constant1/1 -> Sum1/2
  Sum1/1 -> Gain1/1
  Demux/3 -> Sum2/1
  Sum2/1 -> Gain2/1
  Constant2/1 -> Sum2/2
  Gain/1 -> Mux/1
  Sum3/1 -> Gain3/1
  Constant3/1 -> Sum3/2
  Sum5/1 -> Gain/1
  Demux/1 -> Sum5/1
  Gain2/1 -> Mux/3
  Gain3/1 -> Mux/4
  Gain1/1 -> Mux/2
  Demux/2 -> Sum1/1
  Demux/4 -> Sum3/1
  In/1 -> Demux/1
  Mux/1 -> value/1

== system MPC_RL_H2DF/Engine Model2/C2C_NMPC_n1/constraints/Subsystem1 ==
  In : Inport
  Constant : Constant  Value=C2C_NMPC.Normalization.outputs.mean(1)
  Constant1 : Constant  Value=C2C_NMPC.Normalization.outputs.mean(2)
  Constant2 : Constant  Value=C2C_NMPC.Normalization.outputs.mean(3)
  Constant3 : Constant  Value=C2C_NMPC.Normalization.outputs.mean(4)
  Demux : Demux
  Gain : Gain  Gain=1/C2C_NMPC.Normalization.outputs.std(1)
  Gain1 : Gain  Gain=1/C2C_NMPC.Normalization.outputs.std(2)
  Gain2 : Gain  Gain=1/C2C_NMPC.Normalization.outputs.std(3)
  Gain3 : Gain  Gain=1/C2C_NMPC.Normalization.outputs.std(4)
  Mux : Mux
  Sum{1..3,5} (4 alike) : Sum  Inputs=|+-
  ubh_e : Outport
  wires:
  Mux/1 -> ubh_e/1
  In/1 -> Demux/1
  Demux/4 -> Sum3/1
  Demux/2 -> Sum1/1
  Gain1/1 -> Mux/2
  Gain3/1 -> Mux/4
  Gain2/1 -> Mux/3
  Demux/1 -> Sum5/1
  Sum5/1 -> Gain/1
  Constant3/1 -> Sum3/2
  Sum3/1 -> Gain3/1
  Gain/1 -> Mux/1
  Constant2/1 -> Sum2/2
  Sum2/1 -> Gain2/1
  Demux/3 -> Sum2/1
  Sum1/1 -> Gain1/1
  Constant1/1 -> Sum1/2
  Constant/1 -> Sum5/2

== system MPC_RL_H2DF/Engine Model2/C2C_NMPC_n1/constraints/Subsystem2 ==
  In : Inport
  Demux : Demux
  Gain : Gain  Gain=1/C2C_NMPC.Normalization.controls.std(1)
  Gain1 : Gain  Gain=1/C2C_NMPC.Normalization.controls.std(2)
  Gain2 : Gain  Gain=1/C2C_NMPC.Normalization.controls.std(3)
  Gain3 : Gain  Gain=1/C2C_NMPC.Normalization.controls.std(4)
  Mux : Mux
  Out : Outport
  wires:
  Gain/1 -> Mux/1
  Gain2/1 -> Mux/3
  Gain1/1 -> Mux/2
  In/1 -> Demux/1
  Mux/1 -> Out/1
  Demux/1 -> Gain/1
  Demux/2 -> Gain1/1
  Demux/3 -> Gain2/1
  Demux/4 -> Gain3/1
  Gain3/1 -> Mux/4

== system MPC_RL_H2DF/Engine Model2/C2C_NMPC_n1/constraints/Subsystem3 ==
  In : Inport
  Demux : Demux
  Gain : Gain  Gain=1/C2C_NMPC.Normalization.controls.std(1)
  Gain1 : Gain  Gain=1/C2C_NMPC.Normalization.controls.std(2)
  Gain2 : Gain  Gain=1/C2C_NMPC.Normalization.controls.std(3)
  Gain3 : Gain  Gain=1/C2C_NMPC.Normalization.controls.std(4)
  Mux : Mux
  Out : Outport
  wires:
  Gain/1 -> Mux/1
  Gain2/1 -> Mux/3
  Gain1/1 -> Mux/2
  In/1 -> Demux/1
  Mux/1 -> Out/1
  Demux/1 -> Gain/1
  Demux/2 -> Gain1/1
  Demux/3 -> Gain2/1
  Demux/4 -> Gain3/1
  Gain3/1 -> Mux/4

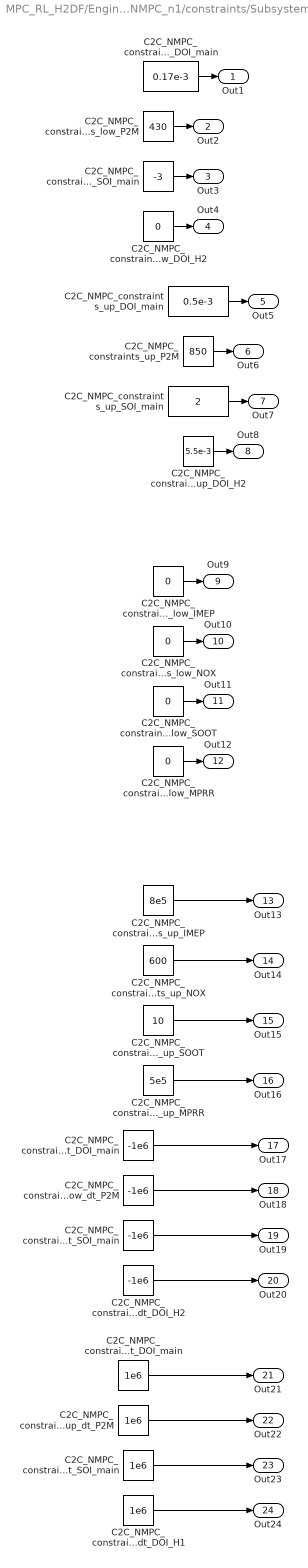
== system MPC_RL_H2DF/Engine Model2/C2C_NMPC_n1/constraints/Subsystem4 ==
  C2C_NMPC_constraints_low_DOI_H2 : Constant  Value=0
  C2C_NMPC_constraints_low_DOI_main : Constant  Value=0.17e-3
  C2C_NMPC_constraints_low_IMEP : Constant  Value=0
  C2C_NMPC_constraints_low_MPRR : Constant  Value=0
  C2C_NMPC_constraints_low_NOX : Constant  Value=0
  C2C_NMPC_constraints_low_P2M : Constant  Value=430
  C2C_NMPC_constraints_low_SOI_main : Constant  Value=-3
  C2C_NMPC_constraints_low_SOOT : Constant  Value=0
  C2C_NMPC_constraints_low_dt_DOI_H2 : Constant  Value=-1e6
  C2C_NMPC_constraints_low_dt_DOI_main : Constant  Value=-1e6
  C2C_NMPC_constraints_low_dt_P2M : Constant  Value=-1e6
  C2C_NMPC_constraints_low_dt_SOI_main : Constant  Value=-1e6
  C2C_NMPC_constraints_up_DOI_H2 : Constant  Value=5.5e-3
  C2C_NMPC_constraints_up_DOI_main : Constant  Value=0.5e-3
  C2C_NMPC_constraints_up_IMEP : Constant  Value=8e5
  C2C_NMPC_constraints_up_MPRR : Constant  Value=5e5
  C2C_NMPC_constraints_up_NOX : Constant  Value=600
  C2C_NMPC_constraints_up_P2M : Constant  Value=850
  C2C_NMPC_constraints_up_SOI_main : Constant  Value=2
  C2C_NMPC_constraints_up_SOOT : Constant  Value=10
  C2C_NMPC_constraints_up_dt_DOI_H1 : Constant  Value=1e6
  C2C_NMPC_constraints_up_dt_DOI_main : Constant  Value=1e6
  C2C_NMPC_constraints_up_dt_P2M : Constant  Value=1e6
  C2C_NMPC_constraints_up_dt_SOI_main : Constant  Value=1e6
  Out1 : Outport
  Out2 : Outport  Port=2
  Out3 : Outport  Port=3
  Out4 : Outport  Port=4
  Out5 : Outport  Port=5
  Out6 : Outport  Port=6
  Out7 : Outport  Port=7
  Out8 : Outport  Port=8
  Out9 : Outport  Port=9
  Out10 : Outport  Port=10
  Out11 : Outport  Port=11
  Out12 : Outport  Port=12
  Out13 : Outport  Port=13
  Out14 : Outport  Port=14
  Out15 : Outport  Port=15
  Out16 : Outport  Port=16
  Out17 : Outport  Port=17
  Out18 : Outport  Port=18
  Out19 : Outport  Port=19
  Out20 : Outport  Port=20
  Out21 : Outport  Port=21
  Out22 : Outport  Port=22
  Out23 : Outport  Port=23
  Out24 : Outport  Port=24
  wires:
  C2C_NMPC_constraints_low_dt_DOI_H2/1 -> Out20/1
  C2C_NMPC_constraints_low_dt_P2M/1 -> Out18/1
  C2C_NMPC_constraints_up_dt_SOI_main/1 -> Out23/1
  C2C_NMPC_constraints_up_dt_DOI_H1/1 -> Out24/1
  C2C_NMPC_constraints_up_DOI_H2/1 -> Out8/1
  C2C_NMPC_constraints_low_dt_DOI_main/1 -> Out17/1
  C2C_NMPC_constraints_low_dt_SOI_main/1 -> Out19/1
  C2C_NMPC_constraints_up_SOOT/1 -> Out15/1
  C2C_NMPC_constraints_up_MPRR/1 -> Out16/1
  C2C_NMPC_constraints_up_NOX/1 -> Out14/1
  C2C_NMPC_constraints_up_IMEP/1 -> Out13/1
  C2C_NMPC_constraints_up_dt_P2M/1 -> Out22/1
  C2C_NMPC_constraints_low_SOI_main/1 -> Out3/1
  C2C_NMPC_constraints_up_dt_DOI_main/1 -> Out21/1
  C2C_NMPC_constraints_low_SOOT/1 -> Out11/1
  C2C_NMPC_constraints_low_DOI_H2/1 -> Out4/1
  C2C_NMPC_constraints_up_P2M/1 -> Out6/1
  C2C_NMPC_constraints_low_P2M/1 -> Out2/1
  C2C_NMPC_constraints_low_DOI_main/1 -> Out1/1
  C2C_NMPC_constraints_low_MPRR/1 -> Out12/1
  C2C_NMPC_constraints_up_SOI_main/1 -> Out7/1
  C2C_NMPC_constraints_up_DOI_main/1 -> Out5/1
  C2C_NMPC_constraints_low_IMEP/1 -> Out9/1
  C2C_NMPC_constraints_low_NOX/1 -> Out10/1

== system MPC_RL_H2DF/Engine Model2/C2C_NMPC_n1/cost_function_weights/Normalize 0 to 1 ==
  In1 : Inport
  Demux : Demux
  Divide{,1..3} (4 alike) : Product  Inputs=*/
  Mux : Mux
  Sum : Sum  Inputs=|++++
  Out1 : Outport
  wires:
  In1/1 -> Demux/1
  Demux/1 -> Sum/1, Divide/1
  Demux/2 -> Divide1/1, Sum/2
  Demux/3 -> Divide2/1, Sum/3
  Demux/4 -> Divide3/1, Sum/4
  Sum/1 -> Divide/2, Divide1/2, Divide2/2, Divide3/2
  Divide3/1 -> Mux/4
  Divide2/1 -> Mux/3
  Divide1/1 -> Mux/2
  Divide/1 -> Mux/1
  Mux/1 -> Out1/1
